simulink model "PumpMotorSim"  (R2025a)
settings: Solver=ode3  StartTime=0.0  StopTime=25  FixedStep=2.5e-5  RelTol=1e-3  AbsTol=1e-3
StartFcn:
  | init_pmsm()
model workspace (MAT data in the model file):
  B = 1
  Tcoul = 1
  k_pump = 1
  p = Simulink.Parameter
  p.Complexity = 'real'
  p.Dimensions = [0 0]
  p.DataType = 'auto'
  x = 1
values from neighbouring files (symbols this model uses):
  B_pump = Simulink.Parameter(B_pump)    [init_pmsm.m]
  K_lambda = 2/(3*p*lambda_m)    (= 4.7619047619)    [init_pmsm.m]
  Ts_ctrl = Simulink.Parameter(Ts_ctrl)    [init_pmsm.m]
  Vdc = Simulink.Parameter(Vdc)    [init_pmsm.m]
undefined symbols (not defined in the file or in its folder): pmsm
libraries: slpidlib x4, mcbeeMathTransformLib x3, mcbcontrollergainlib x2, eePwmGeneratorTwoLevel x2, mcbfoclib x1, mcbpositiondecoderlib x1, mcbcontrolslib x1, spsSVPWMGenerator2LevelLib x1, simulink x1, mcbplantlib x1, spsCurrentMeasurementLib x1, spsDCVoltageSourceLib x1
settings Model: NumberOfSteps=1000  PacingRate=1000  Creator=abrehamtadesse  LastModifiedBy=abrehamtadesse
settings SolverCC: AutoScaleAbsTol=off  AlgebraicLoopSolver=TrustRegion  MaxZcPerStep=1.0
settings DebuggingCC: UnconnectedInputMsg=warning  UnconnectedOutputMsg=warning  UnconnectedLineMsg=warning  SymbolicDimsDataTypeCodeGenerationDiagnostic=none
settings ModelReferenceCC: EnableRefExpFcnMdlSchedulingChecks=on
settings SFSimCC: CustomCodeUndefinedFunction=UseInterfaceOnly
settings RTWCC: GPUComputeCapability=3.5  DLArmComputeVersion=19.05
settings SimscapeCC: SimscapeLogType=all  SimscapeLogSimulationStatistics=on  SimscapeLogDataHistory=10000.0

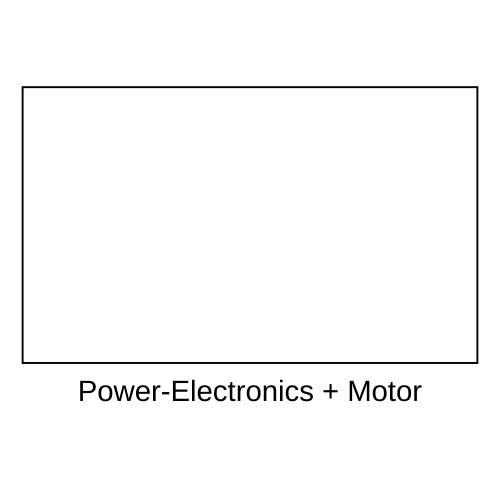
[thumbnail: Simulink's stored preview of the top-level diagram]
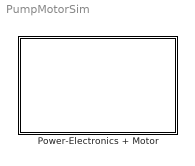
== system PumpMotorSim ==
  Power-Electronics + Motor : Subsystem

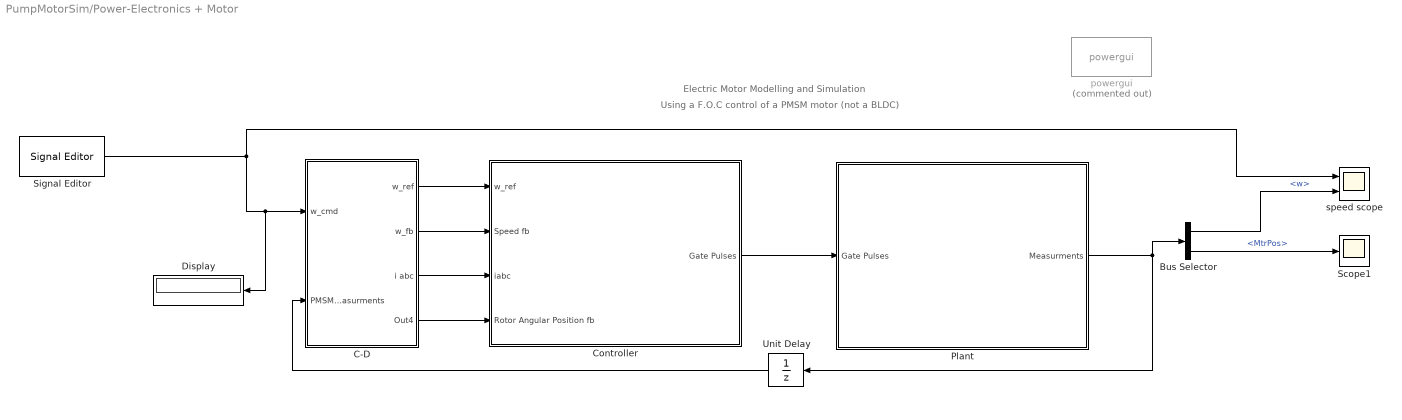
== system PumpMotorSim/Power-Electronics + Motor ==
  note: Using a F.O.C control of a PMSM motor (not a BLDC)
  note: Electric Motor Modelling and Simulation
  Bus Selector : BusSelector  OutputSignals=w,MtrPos
  C-D : Subsystem
  Controller : Subsystem
  Display : Display
  Plant : Subsystem
  Scope1 : Scope
      settings: ActiveDisplayYMinimum=-6.20206329211846  ActiveDisplayYMaximum=8.104243193909431  DataLoggingVariableName=ScopeData3
  Signal Editor : SignalEditorBlockLib/Signal Editor  FileName=untitled.mat  ActiveScenario=Scenario  ActiveSignal=Signal 1  IsBus=off  OutputBusObjectStr=Bus: BusObject  SampleTime=0  ZeroCross=off  OutputAfterFinalValue=Setting to zero  Unit=inherit  PreserveSignalName=on  ApplySigPropsToAllScenarios=on  ApplySigPropsToAllSignals=off  SignalPropertySource=Dialog parameters
  Unit Delay : UnitDelay  SampleTime=-1  HasFrameUpgradeWarning=on
  powergui : spspowerguiLib/powergui  Priority=1  Commented=on  SimulationMode=Continuous  SampleTime=50e-6  frequency=60  Iterations=50  frequencyindice=0  Pbase=100e6  ErrMax=1e-4  UnitsV=kV  UnitsW=MW  buscounter=0  FunctionMessages=off  echomessages=off  EnableUseOfTLC=off  CurrentSourceSwitches=off  DisableSnubberDevices=off  DisableRonSwitches=off  DisableVfSwitches=off  DisplayEquations=off  AutomaticDiscreteSolvers=off  SolverType=Tustin/Backward Euler (TBE)  Interpol=off  ExternalGateDelay=off  methode=off  Ts=100  x0status=blocks  SPID=on  SwTol=0  HookPort=off  NonlinearTolerance=1e-4  nMaxIteration=100  ContinueOnMaxIteration=off  RestoreLinks=warning  ResistiveCurrentMeasurement=off  Frange=[0:2:500]  Ylog=off  Xlog=on  ShowGrid=off  save=off  variable=ZData  structure=0  ZoomFFT=off  StartTime=0.0  cycles=1  DisplayStyle=1  fundamental=60  FreqAxis=off  MaxFrequency=1000  frequencyindicesteady=1  RmsSteady=1  display=off
  speed scope : Scope  NumInputPorts=2
      settings: ActiveDisplayYMinimum=-184.95326256021298  ActiveDisplayYMaximum=1624.3755597064778
  wires:
  Signal Editor/1 -> speed scope/1, Display/1, C-D/1(w_cmd)
  Plant/1(Measurments) -> Bus Selector/1, Unit Delay/1
  Unit Delay/1 -> C-D/2(PMSM_Measurments)
  Controller/1(Gate Pulses) -> Plant/1(Gate Pulses)
  C-D/1(w_ref) -> Controller/1(w_ref)
  C-D/3(i abc) -> Controller/3(iabc)
  C-D/2(w_fb) -> Controller/2(Speed fb)
  C-D/4(Out4) -> Controller/4(Rotor Angular Position fb)
  Bus Selector/2 -> Scope1/1  "<MtrPos>"
  Bus Selector/1 -> speed scope/2  "<w>"

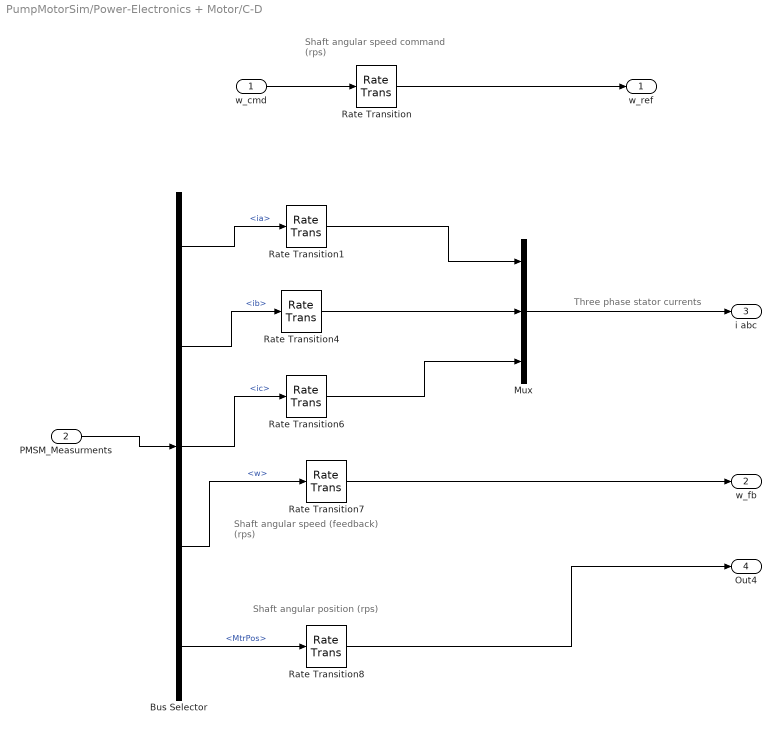
== system PumpMotorSim/Power-Electronics + Motor/C-D ==
  note: Shaft angular speed (feedback) (rps)
  note: Shaft angular position (rps)
  note: Shaft angular speed command (rps)
  note: Three phase stator currents
  w_cmd : Inport
  PMSM_Measurments : Inport  Port=2
  Bus Selector : BusSelector  OutputSignals=ia,ib,ic,w,MtrPos
  Mux : Mux  Inputs=3
  Rate Transition : RateTransition
  Rate Transition{1,4,6..8} (5 alike) : RateTransition  OutPortSampleTimeOpt=Inherit  OutPortSampleTime=0.0001
  w_ref : Outport
  w_fb : Outport  Port=2
  i abc : Outport  Port=3
  Out4 : Outport  Port=4
  wires:
  Rate Transition/1 -> w_ref/1
  w_cmd/1 -> Rate Transition/1
  PMSM_Measurments/1 -> Bus Selector/1
  Bus Selector/1 -> Rate Transition1/1  "<ia>"
  Bus Selector/2 -> Rate Transition4/1  "<ib>"
  Bus Selector/3 -> Rate Transition6/1  "<ic>"
  Bus Selector/4 -> Rate Transition7/1  "<w>"
  Rate Transition4/1 -> Mux/2
  Rate Transition1/1 -> Mux/1
  Mux/1 -> i abc/1
  Rate Transition7/1 -> w_fb/1
  Rate Transition8/1 -> Out4/1
  Bus Selector/5 -> Rate Transition8/1  "<MtrPos>"
  Rate Transition6/1 -> Mux/3

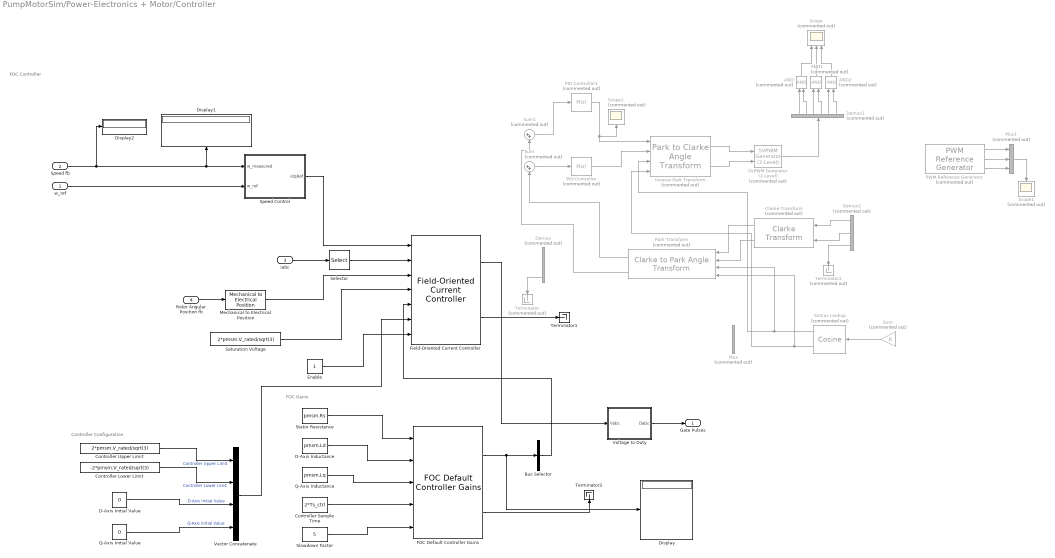
== system PumpMotorSim/Power-Electronics + Motor/Controller ==
  note: FOC Controller
  note: FOC Gains
  note: Controller Configuration
  w_ref : Inport
  Speed fb : Inport  Port=2
  iabc : Inport  Port=3
  Rotor Angular Position fb : Inport  Port=4
  AND : Logic  Commented=on  IconShape=distinctive  AllPortsSameDT=off  OutDataTypeStr=boolean
  AND1 : Logic  Commented=on  IconShape=distinctive  AllPortsSameDT=off  OutDataTypeStr=boolean
  AND2 : Logic  Commented=on  IconShape=distinctive  AllPortsSameDT=off  OutDataTypeStr=boolean
  Bus Selector : BusSelector  OutputSignals=Daxis_Kp,Daxis_Ki*Ts,Qaxis_Kp,Qaxis_Ki*Ts  OutputAsBus=on
  Clarke Transform : mcbeeMathTransformLib/Clarke Transform  Commented=on  VariantControl=Variant2  PowerInvariant=on  UseWithEmbedded=on  PhaseInput=Two inputs
      settings: LibrarySourceBlock=mcbhdllib/Controls/Math Transforms/Clarke Transform
  Controller Lower Limit : Constant  Value=-2*pmsm.V_rated/sqrt(3)
  Controller Sample Time : Constant  Value=2*Ts_ctrl
  Controller Upper Limit : Constant  Value=2*pmsm.V_rated/sqrt(3)  OutDataTypeStr=double
  D-Axis Inductance : Constant  Value=pmsm.Ld
  D-Axis Initial Value : Constant  Value=0
  Demux : Demux  Commented=on  Outputs=3
  Demux1 : Demux  Commented=on  Outputs=6
  Demux2 : Demux  Commented=on  Outputs=3
  Display : Display
  Display1 : Display
  Display2 : Display
  Enable : Constant
  FOC Default Controller Gains : mcbcontrollergainlib/FOC Default Controller Gains  ControllerGainType=Empirical method  motorSelection=PMSM  unitType=SI Unit  outCurrentControlGain=on  outFWCGain=off  outSpeedControlGain=off  externalDelay=off  currentSensorDelay=50e-6  speedSensorDelay=50e-6  speedFilterDelay=0.02
      settings: LibrarySourceBlock=mcblib/Controls/Controllers/FOC Default Controller Gains
  Field-Oriented Current Controller : mcbfoclib/Field-Oriented Current Controller  AngleUnit=Radians  NumberOfLUTPoints=1024  AxisAlignment=D-axis  SaturationMethod=D-Q equivalence  PWMMethod=SPWM: sinusoidal PWM
      settings: LibrarySourceBlock=mcblib/Controls/Controllers/Field-Oriented Current Controller
  Gain : Gain  Commented=on  Gain=6
  Inverse Park Transform : mcbeeMathTransformLib/Park to Clarke Angle Transform  Commented=on  AxisAlignment=D-axis  UseWithEmbedded=on  PhaseInput=Two inputs  ThetaInput=Sine and Cosine electrical position  AngleInput=Per-unit  N_points=1024
      settings: LibrarySourceBlock=mcbhdllib/Controls/Math Transforms/Inverse Park Transform
  Mechanical to Electrical Position : mcbpositiondecoderlib/Mechanical to Electrical Position  PolePairsInputType=Specify via dialog  NrPP=pmsm.p  selectedRange=Radians  MechOfstInputType=Specify via dialog  mechOffsetIn=0  maxAngleIn=2*pi  InputDataType=single  VariantSelect=floating-point
      settings: LibrarySourceBlock=mcblib/Sensor Decoders/Mechanical to Electrical Position
  Mux : Mux  Commented=on  Inputs=2
  Mux1 : Mux  Commented=on  Inputs=3
  PID Controller : slpidlib/PID Controller  Commented=on  Controller=PI  Form=Parallel  TimeDomain=Discrete-time  UseExternalTs=off  SampleTime=.0001  IntegratorMethod=Forward Euler  FilterMethod=Forward Euler  ControllerParametersSource=internal  P=-0.038309  I=0  UseKiTs=off  D=0  UseExternalDerivativeSource=off  N=100  UseFilter=on  TunerSelectOption=Frequency Response Based  InitialConditionSource=internal  InitialConditionForIntegrator=0  InitialConditionForFilter=0  DifferentiatorICPrevScaledInput=0  ExternalReset=none  TrackingMode=off  Kt=1  LimitOutput=off  SatLimitsSource=internal  UpperSaturationLimit=inf  LowerSaturationLimit=-inf  LinearizeAsGain=on  AntiWindupMode=none  Kb=1  LimitIntegrator=off  UpperIntegratorSaturationLimit=inf  LowerIntegratorSaturationLimit=-inf  POutMin=[]  POutMax=[]  IOutMin=[]  IOutMax=[]  DOutMin=[]  DOutMax=[]  NOutMin=[]  NOutMax=[]  SumOutMin=[]  SumOutMax=[]  SaturationOutMin=[]  SaturationOutMax=[]  PParamMin=[]  PParamMax=[]  IParamMin=[]  IParamMax=[]  DParamMin=[]  DParamMax=[]  NParamMin=[]  NParamMax=[]  KbParamMin=[]  KbParamMax=[]  KtParamMin=[]  KtParamMax=[]  KbOutMin=[]  KbOutMax=[]  KtOutMin=[]  KtOutMax=[]  IntegratorOutMin=[]  IntegratorOutMax=[]  FilterOutMin=[]  FilterOutMax=[]  SumI1OutMin=[]  SumI1OutMax=[]  SumI2OutMin=[]  SumI2OutMax=[]  SumI3OutMin=[]  SumI3OutMax=[]  SumI4OutMin=[]  SumI4OutMax=[]  SumDOutMin=[]  SumDOutMax=[]  DifferentiatorOutMin=[]  DifferentiatorOutMax=[]  FilterDiffOutCoefMin=[]  FilterDiffOutCoefMax=[]  ReciprocalOutMin=[]  ReciprocalOutMax=[]  SumDenOutMin=[]  SumDenOutMax=[]  SumNumOutMin=[]  SumNumOutMax=[]  DivideOutMin=[]  DivideOutMax=[]  UdiffTsProdOutMin=[]  UdiffTsProdOutMax=[]  NTsProdOutMin=[]  NTsProdOutMax=[]  UintegralTsProdOutMin=[]  UintegralTsProdOutMax=[]  UngainTsProdOutMin=[]  UngainTsProdOutMax=[]  ClampingZeroOutDataTypeStr=Inherit: Inherit via back propagation  ClampingZeroOutMin=[]  ClampingZeroOutMax=[]  FilterDenConstantOutDataTypeStr=Inherit: Inherit via back propagation  FilterDenConstantOutMin=[]  FilterDenConstantOutMax=[]  PCopyOutDataTypeStr=Inherit: Inherit via back propagation  PCopyOutMin=[]  PCopyOutMax=[]  NCopyOutDataTypeStr=Inherit: Inherit via back propagation  NCopyOutMin=[]  NCopyOutMax=[]  IntegratorContinuousStateAttributes=''  IntegratorStateMustResolveToSignalObject=off  IntegratorRTWStateStorageClass=Auto  FilterContinuousStateAttributes=''  FilterStateMustResolveToSignalObject=off  FilterRTWStateStorageClass=Auto  ParallelPVariant=InternalParameters  IdealPVariant=Disabled  IVariant=InternalParameters  DVariant=Disabled  IntegratorVariant=Discrete  SatVariant=Disabled  AWVariant=Passthrough  PCopyVariant=Disabled  TRVariant=Disabled  FdbkBlocksVariant=Forward  IdealPFdbkVariant=Disabled  SatFdbkVariant=Disabled  DerivativeFilterVariant=Disabled  NVariant=Disabled  NCopyVariant=Disabled_SignalSpec  FilterICVariant=Disabled  IntegratorICVariant=InternalICs  ExternalResetVariant=Disabled  TRSumVariant=Passthrough  SumFdbkVariant=Disabled  SumVariant=Sum_PI  TsampFilterVariant=InternalTs  TsampNgainVariant=Passthrough  TsampIntegralVariant=Disabled_SignalSpec  ExternalSaturationOutDataTypeStr=Inherit: Same as second input  DerivativeSourceVariant=Disabled  PreIntVariant=InternalPreInt
  PID Controller1 : slpidlib/PID Controller  Commented=on  Controller=PI  Form=Parallel  TimeDomain=Discrete-time  UseExternalTs=off  SampleTime=-1  IntegratorMethod=Forward Euler  FilterMethod=Forward Euler  ControllerParametersSource=internal  P=-0.024043  I=-0.015076  UseKiTs=off  D=0  UseExternalDerivativeSource=off  N=100  UseFilter=on  TunerSelectOption=Frequency Response Based  InitialConditionSource=internal  InitialConditionForIntegrator=0  InitialConditionForFilter=0  DifferentiatorICPrevScaledInput=0  ExternalReset=none  TrackingMode=off  Kt=1  LimitOutput=off  SatLimitsSource=internal  UpperSaturationLimit=inf  LowerSaturationLimit=-inf  LinearizeAsGain=on  AntiWindupMode=none  Kb=1  LimitIntegrator=off  UpperIntegratorSaturationLimit=inf  LowerIntegratorSaturationLimit=-inf  POutMin=[]  POutMax=[]  IOutMin=[]  IOutMax=[]  DOutMin=[]  DOutMax=[]  NOutMin=[]  NOutMax=[]  SumOutMin=[]  SumOutMax=[]  SaturationOutMin=[]  SaturationOutMax=[]  PParamMin=[]  PParamMax=[]  IParamMin=[]  IParamMax=[]  DParamMin=[]  DParamMax=[]  NParamMin=[]  NParamMax=[]  KbParamMin=[]  KbParamMax=[]  KtParamMin=[]  KtParamMax=[]  KbOutMin=[]  KbOutMax=[]  KtOutMin=[]  KtOutMax=[]  IntegratorOutMin=[]  IntegratorOutMax=[]  FilterOutMin=[]  FilterOutMax=[]  SumI1OutMin=[]  SumI1OutMax=[]  SumI2OutMin=[]  SumI2OutMax=[]  SumI3OutMin=[]  SumI3OutMax=[]  SumI4OutMin=[]  SumI4OutMax=[]  SumDOutMin=[]  SumDOutMax=[]  DifferentiatorOutMin=[]  DifferentiatorOutMax=[]  FilterDiffOutCoefMin=[]  FilterDiffOutCoefMax=[]  ReciprocalOutMin=[]  ReciprocalOutMax=[]  SumDenOutMin=[]  SumDenOutMax=[]  SumNumOutMin=[]  SumNumOutMax=[]  DivideOutMin=[]  DivideOutMax=[]  UdiffTsProdOutMin=[]  UdiffTsProdOutMax=[]  NTsProdOutMin=[]  NTsProdOutMax=[]  UintegralTsProdOutMin=[]  UintegralTsProdOutMax=[]  UngainTsProdOutMin=[]  UngainTsProdOutMax=[]  ClampingZeroOutDataTypeStr=Inherit: Inherit via back propagation  ClampingZeroOutMin=[]  ClampingZeroOutMax=[]  FilterDenConstantOutDataTypeStr=Inherit: Inherit via back propagation  FilterDenConstantOutMin=[]  FilterDenConstantOutMax=[]  PCopyOutDataTypeStr=Inherit: Inherit via back propagation  PCopyOutMin=[]  PCopyOutMax=[]  NCopyOutDataTypeStr=Inherit: Inherit via back propagation  NCopyOutMin=[]  NCopyOutMax=[]  IntegratorContinuousStateAttributes=''  IntegratorStateMustResolveToSignalObject=off  IntegratorRTWStateStorageClass=Auto  FilterContinuousStateAttributes=''  FilterStateMustResolveToSignalObject=off  FilterRTWStateStorageClass=Auto  ParallelPVariant=InternalParameters  IdealPVariant=Disabled  IVariant=InternalParameters  DVariant=Disabled  IntegratorVariant=Discrete  SatVariant=Disabled  AWVariant=Passthrough  PCopyVariant=Disabled  TRVariant=Disabled  FdbkBlocksVariant=Forward  IdealPFdbkVariant=Disabled  SatFdbkVariant=Disabled  DerivativeFilterVariant=Disabled  NVariant=Disabled  NCopyVariant=Disabled_SignalSpec  FilterICVariant=Disabled  IntegratorICVariant=InternalICs  ExternalResetVariant=Disabled  TRSumVariant=Passthrough  SumFdbkVariant=Disabled  SumVariant=Sum_PI  TsampFilterVariant=InternalTs  TsampNgainVariant=Passthrough  TsampIntegralVariant=Disabled_SignalSpec  ExternalSaturationOutDataTypeStr=Inherit: Same as second input  DerivativeSourceVariant=Disabled  PreIntVariant=InternalPreInt
  PWM Reference Generator : mcbcontrolslib/PWM Reference Generator  Commented=on  inSignal=Valphabeta  modType=SPWM: sinusoidal PWM
      settings: LibrarySourceBlock=mcblib/Controls/Math Transforms/PWM Reference Generator
  Park Transform : mcbeeMathTransformLib/Clarke to Park Angle Transform  Commented=on  AxisAlignment=Q-axis  UseWithEmbedded=on  PhaseInput=Two inputs  ThetaInput=Sine and Cosine electrical position  AngleInput=Per-unit  N_points=1024
      settings: LibrarySourceBlock=mcblib/Controls/Math Transforms/Park Transform
  Q-Axis Inductance : Constant  Value=pmsm.Lq
  Q-Axis Initial Value : Constant  Value=0
  SVPWM Generator (2-Level) : spsSVPWMGenerator2LevelLib/SVPWM Generator (2-Level)  Commented=on  InputType=alpha-beta components  SwitchingPattern=Pattern #2  Fc=1e5  ParUref=[0.8 -30 50]  Ts=1/1e5
  Saturation Voltage : Constant  Value=2*pmsm.V_rated/sqrt(3)
  Scope : Scope  Commented=on  NumInputPorts=3
      settings: ActiveDisplayString=3  ActiveDisplayYMinimum=0.035067000175810326  ActiveDisplayYMaximum=1.1147617896359672  DataLoggingVariableName=ScopeData2
  Scope1 : Scope  Commented=on
      settings: ActiveDisplayYMinimum=-428.41416338659832  ActiveDisplayYMaximum=298.358637517937  DataLoggingVariableName=ScopeData4
  Scope2 : Scope  Commented=on
      settings: ActiveDisplayYMinimum=-2.8132759811039056  ActiveDisplayYMaximum=22.715520133300725  DataLoggingVariableName=ScopeData6
  Selector : Selector  InputPortWidth=3  IndexOptions=Index vector (dialog)  Indices=[1 2]  OutputSizes=1
  SinCos Lookup : simulink/Lookup Tables/Cosine  Commented=on  Formula=sin(2*pi*u) and cos(2*pi*u)  NumDataPoints=(2^5)+1  OutputWordLength=16  InternalRulePriority=Speed
      settings: LibrarySourceBlock=|
      | simulink/Quick Insert/Lookup
      | Tables/SinCos Lookup
  Slowdown Factor : Constant  Value=5
  Speed Control : Subsystem
  Stator Resistance : Constant  Value=pmsm.Rs
  Sum : Sum  Commented=on  Inputs=|++
  Sum1 : Sum  Commented=on  Inputs=|++
  Terminator : Terminator  Commented=on
  Terminator1 : Terminator
  Terminator2 : Terminator  Commented=on
  Terminator3 : Terminator
  Vector Concatenate : Concatenate  NumInputs=4
  Voltage to Duty : Subsystem
  Gate Pulses : Outport
  wires:
  Gain/1 -> SinCos Lookup/1
  SinCos Lookup/1 -> Inverse Park Transform/3, Park Transform/3
  SinCos Lookup/2 -> Inverse Park Transform/4, Park Transform/4
  SVPWM Generator (2-Level)/1 -> Demux1/1
  w_ref/1 -> Speed Control/2(w_ref)
  Clarke Transform/1 -> Park Transform/1
  Demux/3 -> Terminator/1
  Demux2/1 -> Clarke Transform/1
  Demux2/2 -> Clarke Transform/2
  Demux2/3 -> Terminator2/1
  Clarke Transform/2 -> Park Transform/2
  PWM Reference Generator/1 -> Mux1/1
  PWM Reference Generator/2 -> Mux1/2
  PWM Reference Generator/3 -> Mux1/3
  Mux1/1 -> Scope1/1
  Inverse Park Transform/1 -> SVPWM Generator (2-Level)/1
  Inverse Park Transform/2 -> SVPWM Generator (2-Level)/2
  AND/1 -> Scope/1
  AND1/1 -> Scope/2
  AND2/1 -> Scope/3
  Demux1/1 -> AND/1
  Demux1/2 -> AND/2
  Demux1/3 -> AND1/1
  Demux1/4 -> AND1/2
  Demux1/5 -> AND2/1
  Demux1/6 -> AND2/2
  Park Transform/2 -> Sum1/2
  Park Transform/1 -> Sum/2
  PID Controller/1 -> Inverse Park Transform/2
  Sum/1 -> PID Controller/1
  PID Controller1/1 -> Scope2/1, Inverse Park Transform/1
  Sum1/1 -> PID Controller1/1
  Speed Control/1(idqRef) -> Field-Oriented Current Controller/1
  iabc/1 -> Selector/1
  Rotor Angular Position fb/1 -> Mechanical to Electrical Position/1
  Mechanical to Electrical Position/1 -> Field-Oriented Current Controller/3
  Saturation Voltage/1 -> Field-Oriented Current Controller/4
  Controller Sample Time/1 -> FOC Default Controller Gains/4
  Slowdown Factor/1 -> FOC Default Controller Gains/5
  Stator Resistance/1 -> FOC Default Controller Gains/1
  D-Axis Inductance/1 -> FOC Default Controller Gains/2
  Q-Axis Inductance/1 -> FOC Default Controller Gains/3
  FOC Default Controller Gains/1 -> Display/1, Bus Selector/1
  Bus Selector/1 -> Field-Oriented Current Controller/5
  Controller Upper Limit/1 -> Vector Concatenate/1  "Controller Upper Limit"
  Controller Lower Limit/1 -> Vector Concatenate/2  "Controller Lower Limit"
  D-Axis Initial Value/1 -> Vector Concatenate/3  "D-Axis Initial Value"
  Q-Axis Initial Value/1 -> Vector Concatenate/4  "Q-Axis Initial Value"
  Vector Concatenate/1 -> Field-Oriented Current Controller/6
  Enable/1 -> Field-Oriented Current Controller/7
  Field-Oriented Current Controller/1 -> Voltage to Duty/1(Vabc)
  Voltage to Duty/1(Dabc) -> Gate Pulses/1
  Field-Oriented Current Controller/2 -> Terminator1/1
  FOC Default Controller Gains/2 -> Terminator3/1
  Speed fb/1 -> Display1/1, Speed Control/1(w_measured), Display2/1
  Selector/1 -> Field-Oriented Current Controller/2

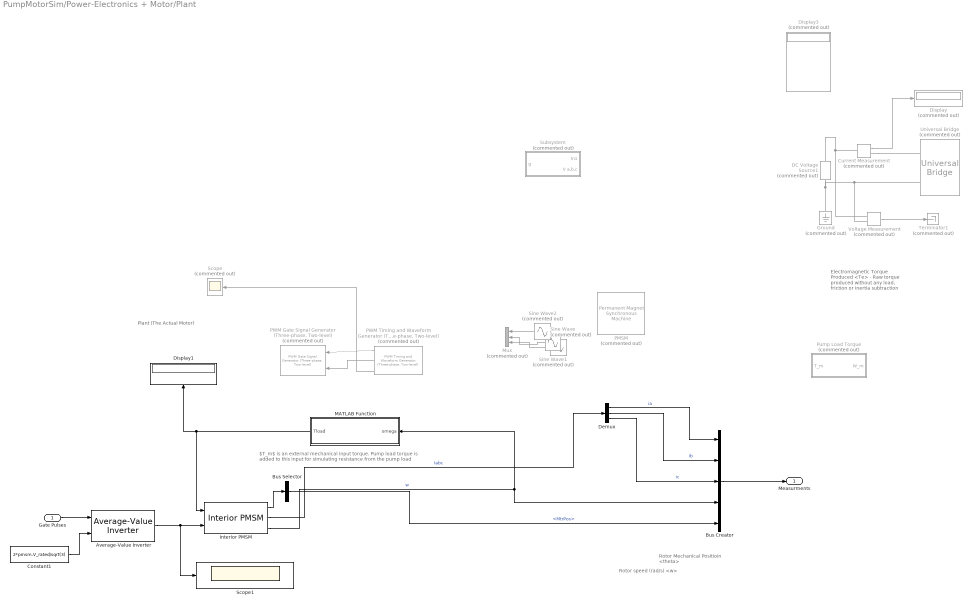
== system PumpMotorSim/Power-Electronics + Motor/Plant ==
  note: Electromagnetic Torque Produced <Te>
      | - Raw torque produced without any load,
      | friction or inertia subtraction
  note: Rotor speed (rad/s) <w>
  note: Rotor Mechanical Positioin <theta>
  note: Plant (The Actual Motor)
  note: $T_m$ is an external mechanical input torque. Pump load torque is added to this input
      | for simulating resistance from the pump load
  Gate Pulses : Inport
  Average-Value Inverter : mcbplantlib/Average-Value Inverter
      settings: LibrarySourceBlock=mcblib/Electrical Systems/Inverters/Average-Value Inverter
  Bus Creator : BusCreator  Inputs=5
  Bus Selector : BusSelector  OutputSignals=MtrPos
  Constant1 : Constant  Value=2*pmsm.V_rated/sqrt(3)
  Current Measurement : spsCurrentMeasurementLib/Current Measurement  Commented=on  PhasorSimulation=off  OutputType=Complex  PSBequivalent=0
  DC Voltage Source1 : spsDCVoltageSourceLib/DC Voltage Source  Commented=on  Amplitude=100  Measurements=Voltage
  Demux : Demux  Outputs=3
  Display : Display  Commented=on
  Display1 : Display
  Display3 : Display  Commented=on
  Ground : spsGroundLib/Ground  Commented=on  LConnTagsString=a
  Interior PMSM : autolibpmsminterior/Interior PMSM  port_config=Torque  sim_type=Discrete  Ts=Ts_ctrl  P=pmsm.p  Rs=pmsm.Rs  Ldq=[pmsm.Ld, pmsm.Lq]  KConstText=Permanent flux linkage constant (lambda_pm):  lambda_pm=lambda_m  Ke=159.9771  mechanical=[pmsm.J, 0, 0]  idq0=[0 0]  theta_init=0  omega_init=0  KConst=pmsm.FluxPM  lambda_pm_calc=pmsm.FluxPM  Kt=0.07  RefBlkName='autolibpmsminterior/Interior PMSM'  aMode=5
      settings: LibrarySourceBlock=mcblib/Electrical Systems/Motors/Interior PMSM
  MATLAB Function : MATLAB Function  TreatAsAtomicUnit=on
  Mux : Mux  Commented=on  Inputs=3
  PMSM : spsPermanentMagnetSynchronousMachineLib/Permanent Magnet Synchronous Machine  Commented=on  NbPhases=3  FluxDistribution=Sinusoidal  RotorType=Round  MechanicalLoad=Torque Tm  PresetModel=No  ShowDetailedParameters=on  MeasurementBus=on  Resistance=0.18  Inductance=8.5e-3  dqInductances=[8.5e-3,8.5e-3]  La=0.000835  MachineConstant=Flux linkage established by magnets (V.s)  Flux=0.0714394  VoltageCst=51.8307  TorqueCst=0.42864  Flat=120  Mechanical=[0.000621417 0.000303448 4]  PolePairs=4  InitialConditions=[0,0, 0,0]  InitialConditions5ph=[0 0 0 0 0 0]  RefAngle=90 degrees behind phase A axis (modified Park)  IterativeDiscreteModel=Trapezoidal non iterative  TsBlock=-1  TsPowergui=0
  "PWM Gate Signal Generator (Three-phase, Two-level)" : eePwmGeneratorTwoLevel/PWM Gate Signal Generator (Three-phase, Two-level)  Commented=on  fsw=1e3  Ts=1e-05
      settings: SamplingMode=Natural
      settings: LibrarySourceBlock=|
      | ee_sl_lib/Pulse Width
      | Modulation/PWM Gate Signal Generator
      | (Three-phase, Two-level)
  "PWM Timing and Waveform Generator (Three-phase, Two-level)" : eePwmGeneratorTwoLevel/PWM Timing and Waveform Generator (Three-phase, Two-level)  Commented=on  PWMMode=Continuous PWM (CPWM)  CPWMMode=SPWM: sinusoidal PWM  DPWMMode=60 DPWM (-30 degree shift): -30 degree shift from 60 DPWM  fsw=1e3
      settings: SamplingMode=Natural
      settings: LibrarySourceBlock=|
      | ee_sl_lib/Pulse Width
      | Modulation/PWM Timing and Waveform
      | Generator
      | (Three-phase, Two-level)
  Pump Load Torque : Subsystem  Commented=on
  Scope : Scope  Commented=on
      settings: ActiveDisplayYMinimum=-1.25  ActiveDisplayYMaximum=1.25
  Scope1 : Scope
      settings: ActiveDisplayYMinimum=-83.281413167694254  ActiveDisplayYMaximum=153.56093098145351  DataLoggingVariableName=ScopeData7
  Sine Wave : Sin  Commented=on  Phase=2*pi/3  SampleTime=0
  Sine Wave1 : Sin  Commented=on  Phase=-2*pi/3  SampleTime=0
  Sine Wave2 : Sin  Commented=on  SampleTime=0
  Subsystem : Subsystem  Commented=on
  Terminator1 : Terminator  Commented=on
  Universal Bridge : spsUniversalBridgeLib/Universal Bridge  Commented=on  Arms=3  SnubberResistance=1e5  SnubberCapacitance=inf  Device=MOSFET / Diodes  Ron=1e-3  Lon=0  ForwardVoltages="[  0  0  ]"  ForwardVoltage=0  GTOparameters=[ 10e-6 , 20e-6 ]  IGBTparameters=[ 1e-6 , 2e-6 ]  Measurements=All voltages and currents  Measurements_2=None  converterType=Rectifier
  Voltage Measurement : spsVoltageMeasurementLib/Voltage Measurement  Commented=on  PhasorSimulation=off  OutputType=Complex  PSBequivalent=0
  Measurments : Outport
  wires:
  Bus Creator/1 -> Measurments/1
  Demux/1 -> Bus Creator/1  "ia"
  Demux/2 -> Bus Creator/2  "ib"
  Demux/3 -> Bus Creator/3  "ic"
  Current Measurement/1 -> Display/1
  "PWM Timing and Waveform Generator (Three-phase, Two-level)"/1 -> "PWM Gate Signal Generator (Three-phase, Two-level)"/1
  "PWM Timing and Waveform Generator (Three-phase, Two-level)"/2 -> "PWM Gate Signal Generator (Three-phase, Two-level)"/2
  "PWM Timing and Waveform Generator (Three-phase, Two-level)"/3 -> Scope/1
  Sine Wave2/1 -> Mux/1
  Sine Wave1/1 -> Mux/2
  Sine Wave/1 -> Mux/3
  Voltage Measurement/1 -> Terminator1/1
  Gate Pulses/1 -> Average-Value Inverter/1
  Constant1/1 -> Average-Value Inverter/2
  MATLAB Function/1(Tload) -> Display1/1, Interior PMSM/1
  Average-Value Inverter/1 -> Scope1/1, Interior PMSM/2
  Interior PMSM/2 -> Demux/1  "Iabc"
  Interior PMSM/1 -> Bus Selector/1
  Interior PMSM/3 -> MATLAB Function/1(omega), Bus Creator/4  "w"
  Bus Selector/1 -> Bus Creator/5  "<MtrPos>"
  connections:
  Current Measurement/RConn1 -- Universal Bridge/RConn1
  DC Voltage Source1/LConn1 -- Ground/LConn1 -- Voltage Measurement/LConn2 -- Universal Bridge/RConn2
  DC Voltage Source1/RConn1 -- Voltage Measurement/LConn1 -- Current Measurement/LConn1

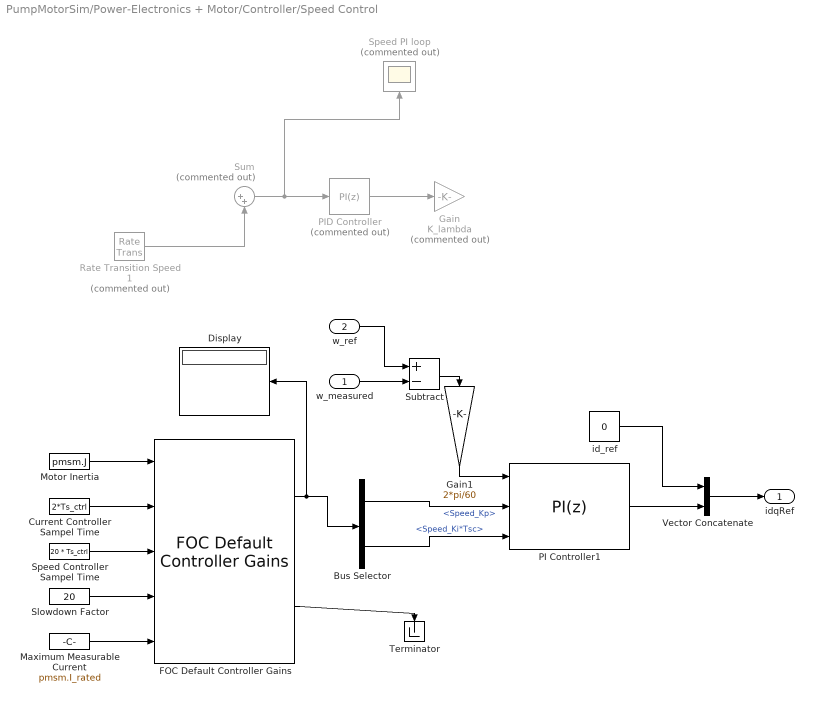
== system PumpMotorSim/Power-Electronics + Motor/Controller/Speed Control ==
  w_measured : Inport
  w_ref : Inport  Port=2
  Bus Selector : BusSelector  OutputSignals=Speed_Kp,Speed_Ki*Tsc
  Current Controller Sampel Time : Constant  Value=2*Ts_ctrl
  Display : Display
  FOC Default Controller Gains : mcbcontrollergainlib/FOC Default Controller Gains  ControllerGainType=Empirical method  motorSelection=PMSM  unitType=SI Unit  outCurrentControlGain=off  outFWCGain=off  outSpeedControlGain=on  externalDelay=off  currentSensorDelay=50e-6  speedSensorDelay=50e-6  speedFilterDelay=0.02
      settings: LibrarySourceBlock=mcblib/Controls/Controllers/FOC Default Controller Gains
  Gain : Gain  Commented=on  Gain=K_lambda
  Gain1 : Gain  Gain=2*pi/60
  Maximum Measurable Current : Constant  Value=pmsm.I_rated
  Motor Inertia : Constant  Value=pmsm.J
  PI Controller1 : slpidlib/PID Controller  Controller=PI  Form=Parallel  TimeDomain=Discrete-time  UseExternalTs=off  SampleTime=-1  IntegratorMethod=Forward Euler  FilterMethod=Forward Euler  ControllerParametersSource=external  P=1  I=1  UseKiTs=on  D=0  UseExternalDerivativeSource=off  N=100  UseFilter=on  TunerSelectOption=Transfer Function Based (PID Tuner App)  InitialConditionSource=internal  InitialConditionForIntegrator=0  InitialConditionForFilter=0  DifferentiatorICPrevScaledInput=0  ExternalReset=none  TrackingMode=off  Kt=1  LimitOutput=on  SatLimitsSource=internal  UpperSaturationLimit=pmsm.I_rated  LowerSaturationLimit=-pmsm.I_rated  LinearizeAsGain=on  AntiWindupMode=clamping  Kb=1  LimitIntegrator=on  UpperIntegratorSaturationLimit=pmsm.I_rated  LowerIntegratorSaturationLimit=-pmsm.I_rated  RndMeth=Simplest  POutMin=[]  POutMax=[]  IOutMin=[]  IOutMax=[]  DOutMin=[]  DOutMax=[]  NOutMin=[]  NOutMax=[]  SumOutMin=[]  SumOutMax=[]  SaturationOutDataTypeStr=Inherit: Inherit via back propagation  SaturationOutMin=[]  SaturationOutMax=[]  PParamMin=[]  PParamMax=[]  IParamMin=[]  IParamMax=[]  DParamMin=[]  DParamMax=[]  NParamMin=[]  NParamMax=[]  KbParamMin=[]  KbParamMax=[]  KtParamMin=[]  KtParamMax=[]  KbOutMin=[]  KbOutMax=[]  KtOutMin=[]  KtOutMax=[]  IntegratorOutMin=[]  IntegratorOutMax=[]  FilterOutMin=[]  FilterOutMax=[]  SumI1OutMin=[]  SumI1OutMax=[]  SumI2OutMin=[]  SumI2OutMax=[]  SumI3OutMin=[]  SumI3OutMax=[]  SumI4OutMin=[]  SumI4OutMax=[]  SumDOutMin=[]  SumDOutMax=[]  DifferentiatorOutMin=[]  DifferentiatorOutMax=[]  FilterDiffOutCoefMin=[]  FilterDiffOutCoefMax=[]  ReciprocalOutMin=[]  ReciprocalOutMax=[]  SumDenOutMin=[]  SumDenOutMax=[]  SumNumOutMin=[]  SumNumOutMax=[]  DivideOutMin=[]  DivideOutMax=[]  UdiffTsProdOutMin=[]  UdiffTsProdOutMax=[]  NTsProdOutMin=[]  NTsProdOutMax=[]  UintegralTsProdOutMin=[]  UintegralTsProdOutMax=[]  UngainTsProdOutMin=[]  UngainTsProdOutMax=[]  ClampingZeroOutDataTypeStr=Inherit: Inherit via back propagation  ClampingZeroOutMin=[]  ClampingZeroOutMax=[]  FilterDenConstantOutDataTypeStr=Inherit: Inherit via back propagation  FilterDenConstantOutMin=[]  FilterDenConstantOutMax=[]  PCopyOutDataTypeStr=Inherit: Inherit via back propagation  PCopyOutMin=[]  PCopyOutMax=[]  NCopyOutDataTypeStr=Inherit: Inherit via back propagation  NCopyOutMin=[]  NCopyOutMax=[]  IntegratorContinuousStateAttributes=''  IntegratorStateMustResolveToSignalObject=off  IntegratorRTWStateStorageClass=Auto  FilterContinuousStateAttributes=''  FilterStateMustResolveToSignalObject=off  FilterRTWStateStorageClass=Auto  ParallelPVariant=ExternalParameters  IdealPVariant=Disabled  IVariant=ExternalParameters  DVariant=Disabled  IntegratorVariant=Discrete  SatVariant=Enabled  AWVariant=DiscClampingParallel  PCopyVariant=Disabled  TRVariant=Disabled  FdbkBlocksVariant=Forward  IdealPFdbkVariant=Disabled  SatFdbkVariant=Disabled  DerivativeFilterVariant=Disabled  NVariant=Disabled  NCopyVariant=Disabled_SignalSpec  FilterICVariant=Disabled  IntegratorICVariant=InternalICs  ExternalResetVariant=Disabled  TRSumVariant=Passthrough  SumFdbkVariant=Disabled  SumVariant=Sum_PI  TsampFilterVariant=InternalTs  TsampNgainVariant=Passthrough  TsampIntegralVariant=Disabled_SignalSpec  ExternalSaturationOutDataTypeStr=Inherit: Same as second input  DerivativeSourceVariant=Disabled  PreIntVariant=InternalPreInt
      settings: LibrarySourceBlock=mcblib/Controls/Controllers/PI Controller
  PID Controller : slpidlib/PID Controller  Commented=on  Controller=PI  Form=Parallel  TimeDomain=Discrete-time  UseExternalTs=off  SampleTime=-1  IntegratorMethod=Forward Euler  FilterMethod=Forward Euler  ControllerParametersSource=internal  P=-0.23505  I=0  UseKiTs=off  D=0  UseExternalDerivativeSource=off  N=100  UseFilter=on  TunerSelectOption=Frequency Response Based  InitialConditionSource=internal  InitialConditionForIntegrator=0  InitialConditionForFilter=0  DifferentiatorICPrevScaledInput=0  ExternalReset=none  TrackingMode=off  Kt=1  LimitOutput=off  SatLimitsSource=internal  UpperSaturationLimit=inf  LowerSaturationLimit=-inf  LinearizeAsGain=on  AntiWindupMode=none  Kb=1  LimitIntegrator=off  UpperIntegratorSaturationLimit=inf  LowerIntegratorSaturationLimit=-inf  POutMin=[]  POutMax=[]  IOutMin=[]  IOutMax=[]  DOutMin=[]  DOutMax=[]  NOutMin=[]  NOutMax=[]  SumOutMin=[]  SumOutMax=[]  SaturationOutMin=[]  SaturationOutMax=[]  PParamMin=[]  PParamMax=[]  IParamMin=[]  IParamMax=[]  DParamMin=[]  DParamMax=[]  NParamMin=[]  NParamMax=[]  KbParamMin=[]  KbParamMax=[]  KtParamMin=[]  KtParamMax=[]  KbOutMin=[]  KbOutMax=[]  KtOutMin=[]  KtOutMax=[]  IntegratorOutMin=[]  IntegratorOutMax=[]  FilterOutMin=[]  FilterOutMax=[]  SumI1OutMin=[]  SumI1OutMax=[]  SumI2OutMin=[]  SumI2OutMax=[]  SumI3OutMin=[]  SumI3OutMax=[]  SumI4OutMin=[]  SumI4OutMax=[]  SumDOutMin=[]  SumDOutMax=[]  DifferentiatorOutMin=[]  DifferentiatorOutMax=[]  FilterDiffOutCoefMin=[]  FilterDiffOutCoefMax=[]  ReciprocalOutMin=[]  ReciprocalOutMax=[]  SumDenOutMin=[]  SumDenOutMax=[]  SumNumOutMin=[]  SumNumOutMax=[]  DivideOutMin=[]  DivideOutMax=[]  UdiffTsProdOutMin=[]  UdiffTsProdOutMax=[]  NTsProdOutMin=[]  NTsProdOutMax=[]  UintegralTsProdOutMin=[]  UintegralTsProdOutMax=[]  UngainTsProdOutMin=[]  UngainTsProdOutMax=[]  ClampingZeroOutDataTypeStr=Inherit: Inherit via back propagation  ClampingZeroOutMin=[]  ClampingZeroOutMax=[]  FilterDenConstantOutDataTypeStr=Inherit: Inherit via back propagation  FilterDenConstantOutMin=[]  FilterDenConstantOutMax=[]  PCopyOutDataTypeStr=Inherit: Inherit via back propagation  PCopyOutMin=[]  PCopyOutMax=[]  NCopyOutDataTypeStr=Inherit: Inherit via back propagation  NCopyOutMin=[]  NCopyOutMax=[]  IntegratorContinuousStateAttributes=''  IntegratorStateMustResolveToSignalObject=off  IntegratorRTWStateStorageClass=Auto  FilterContinuousStateAttributes=''  FilterStateMustResolveToSignalObject=off  FilterRTWStateStorageClass=Auto  ParallelPVariant=InternalParameters  IdealPVariant=Disabled  IVariant=InternalParameters  DVariant=Disabled  IntegratorVariant=Discrete  SatVariant=Disabled  AWVariant=Passthrough  PCopyVariant=Disabled  TRVariant=Disabled  FdbkBlocksVariant=Forward  IdealPFdbkVariant=Disabled  SatFdbkVariant=Disabled  DerivativeFilterVariant=Disabled  NVariant=Disabled  NCopyVariant=Disabled_SignalSpec  FilterICVariant=Disabled  IntegratorICVariant=InternalICs  ExternalResetVariant=Disabled  TRSumVariant=Passthrough  SumFdbkVariant=Disabled  SumVariant=Sum_PI  TsampFilterVariant=InternalTs  TsampNgainVariant=Passthrough  TsampIntegralVariant=Disabled_SignalSpec  ExternalSaturationOutDataTypeStr=Inherit: Same as second input  DerivativeSourceVariant=Disabled  PreIntVariant=InternalPreInt
  Rate Transition Speed 1 : RateTransition  Commented=on  OutPortSampleTime=0.0001
  Slowdown Factor : Constant  Value=20
  Speed Controller Sampel Time : Constant  Value=20 * Ts_ctrl
  Speed PI loop : Scope  Commented=on
      settings: ActiveDisplayYMinimum=-244.4857534645582  ActiveDisplayYMaximum=475.64873955619373  DataLoggingVariableName=ScopeData5
  Subtract : Sum  Inputs=+-
  Sum : Sum  Commented=on  Inputs=|++
  Terminator : Terminator
  Vector Concatenate : Concatenate
  id_ref : Constant  Value=0
  idqRef : Outport
  wires:
  Rate Transition Speed 1/1 -> Sum/2
  PID Controller/1 -> Gain/1
  Sum/1 -> PID Controller/1, Speed PI loop/1
  Motor Inertia/1 -> FOC Default Controller Gains/1
  Current Controller Sampel Time/1 -> FOC Default Controller Gains/2
  Speed Controller Sampel Time/1 -> FOC Default Controller Gains/3
  Slowdown Factor/1 -> FOC Default Controller Gains/4
  Maximum Measurable Current/1 -> FOC Default Controller Gains/5
  FOC Default Controller Gains/1 -> Display/1, Bus Selector/1
  Bus Selector/1 -> PI Controller1/2  "<Speed_Kp>"
  Bus Selector/2 -> PI Controller1/3  "<Speed_Ki*Tsc>"
  w_ref/1 -> Subtract/1
  w_measured/1 -> Subtract/2
  id_ref/1 -> Vector Concatenate/1
  PI Controller1/1 -> Vector Concatenate/2
  Vector Concatenate/1 -> idqRef/1
  FOC Default Controller Gains/2 -> Terminator/1
  Subtract/1 -> Gain1/1
  Gain1/1 -> PI Controller1/1

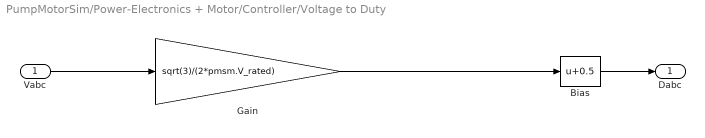
== system PumpMotorSim/Power-Electronics + Motor/Controller/Voltage to Duty ==
  Vabc : Inport
  Bias : Bias  Bias=0.5  SaturateOnIntegerOverflow=off
  Gain : Gain  Gain=sqrt(3)/(2*pmsm.V_rated)
  Dabc : Outport
  wires:
  Gain/1 -> Bias/1
  Bias/1 -> Dabc/1
  Vabc/1 -> Gain/1

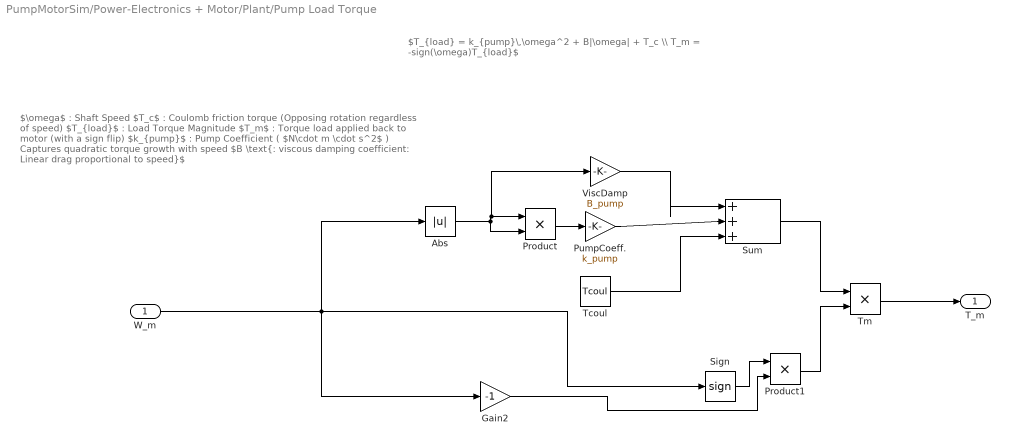
== system PumpMotorSim/Power-Electronics + Motor/Plant/Pump Load Torque ==
  note: $\omega$ : Shaft Speed
      | $T_c$ : Coulomb friction torque (Opposing rotation regardless of speed)
      | $T_{load}$ : Load Torque Magnitude
      | $T_m$ : Torque load applied back to motor (with a sign flip)
      | $k_{pump}$ : Pump Coefficient ( $N\cdot m \cdot s^2$ ) Captures quadratic torque growth with speed
      | $B \text{: viscous damping coefficient: Linear drag proportional to speed}$
  note: $T_{load} = k_{pump}\,\omega^2 + B|\omega| + T_c \\ T_m = -sign(\omega)T_{load}$
  W_m : Inport
  Abs : Abs  SaturateOnIntegerOverflow=off
  Gain2 : Gain  Gain=-1
  Product : Product
  Product1 : Product
  PumpCoeff. : Gain  Gain=k_pump
  Sign : Signum
  Sum : Sum  Inputs=|+++
  Tcoul : Constant  Value=Tcoul
  Tm : Product
  ViscDamp : Gain  Gain=B_pump
  T_m : Outport
  wires:
  Abs/1 -> ViscDamp/1, Product/1, Product/2
  Product/1 -> PumpCoeff./1
  PumpCoeff./1 -> Sum/2
  Tcoul/1 -> Sum/3
  ViscDamp/1 -> Sum/1
  Sign/1 -> Product1/1
  Gain2/1 -> Product1/2
  Sum/1 -> Tm/1
  Product1/1 -> Tm/2
  Tm/1 -> T_m/1
  W_m/1 -> Abs/1, Sign/1, Gain2/1

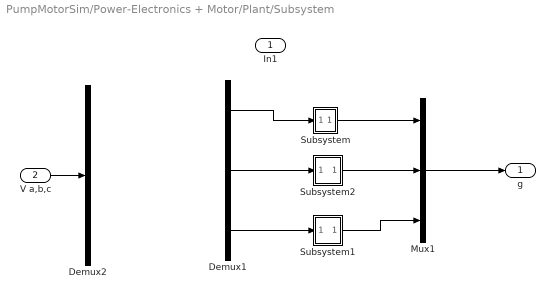
== system PumpMotorSim/Power-Electronics + Motor/Plant/Subsystem ==
  In1 : Inport
  V a,b,c : Inport  Port=2
  Demux1 : Demux  Outputs=3
  Demux2 : Demux  Outputs=3
  Mux1 : Mux  Inputs=3
  Subsystem : Subsystem
  Subsystem1 : Subsystem
  Subsystem2 : Subsystem
  g : Outport
  wires:
  Subsystem/1(Out1) -> Mux1/1
  Demux1/1 -> Subsystem/1(In1)
  Demux1/2 -> Subsystem2/1(In1)
  Demux1/3 -> Subsystem1/1(In1)
  Subsystem2/1(Out1) -> Mux1/2
  Subsystem1/1(Out1) -> Mux1/3
  Mux1/1 -> g/1
  V a,b,c/1 -> Demux2/1

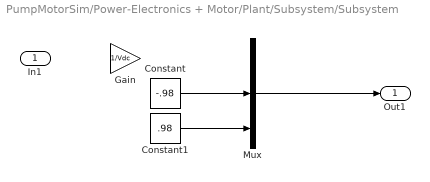
== system PumpMotorSim/Power-Electronics + Motor/Plant/Subsystem/Subsystem ==
  In1 : Inport
  Constant : Constant  Value=-.98
  Constant1 : Constant  Value=.98
  Gain : Gain  Gain=1/Vdc
  Mux : Mux  Inputs=3
  Out1 : Outport
  wires:
  Constant/1 -> Mux/2
  Constant1/1 -> Mux/3
  Mux/1 -> Out1/1

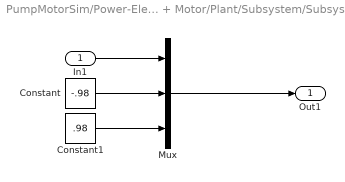
== system PumpMotorSim/Power-Electronics + Motor/Plant/Subsystem/Subsystem1 ==
  In1 : Inport
  Constant : Constant  Value=-.98
  Constant1 : Constant  Value=.98
  Mux : Mux  Inputs=3
  Out1 : Outport
  wires:
  In1/1 -> Mux/1
  Constant/1 -> Mux/2
  Constant1/1 -> Mux/3
  Mux/1 -> Out1/1

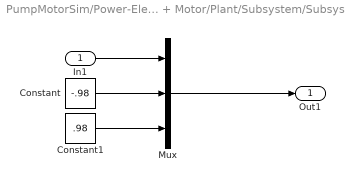
== system PumpMotorSim/Power-Electronics + Motor/Plant/Subsystem/Subsystem2 ==
  In1 : Inport
  Constant : Constant  Value=-.98
  Constant1 : Constant  Value=.98
  Mux : Mux  Inputs=3
  Out1 : Outport
  wires:
  In1/1 -> Mux/1
  Constant/1 -> Mux/2
  Constant1/1 -> Mux/3
  Mux/1 -> Out1/1

== matlab function PumpMotorSim/Power-Electronics + Motor/Plant/MATLAB Function ==
  data: omega input; Tload output
function Tload = pump_load(omega)
% Passive, smooth pump/shaft load (SI units)
% omega [rad/s] → Tload [N·m], always resists motion

Kq   = 3e-5;   % quadratic drag  [N·m/(rad/s)^2]
B    = 2e-4;   % viscous friction [N·m·s/rad]
Tc   = 1e-2;   % Coulomb friction [N·m]
epsw = 1e-3;   % smoothing speed  [rad/s]
Tmax = 3.0;    % safety clamp     [N·m], ~2–3× rated

Tdrag = Kq * omega .* abs(omega);            % ω|ω|
Tvisc = B  * omega;                          % Bω
Tcoul = Tc * tanh(omega/epsw);               % smooth sign(ω)

Tload = Tdrag + Tvisc + Tcoul;               % ≥ 0 in magnitude
Tload = min(max(Tload, -Tmax), Tmax);        % clamp
end
